simulink model "Test_Byte_Demultiplexer_1_to_4"  (Simulink 8.1)
settings: Solver=ode45  StartTime=0.0  StopTime=len  RelTol=1e-3
libraries: Byte_Demultiplexers_Lib x1, commutil2 x1
settings Model: Creator=N  LastModifiedBy=uzivatel
settings DataIOCC: LimitDataPoints=off  SignalLoggingSaveFormat=Dataset
settings OptimizationCC: ExpressionDepthLimit=128
settings DebuggingCC: UnderspecifiedInitializationDetection=Simplified  MergeDetectMultiDrivingBlocksExec=error  SolverPrmCheckMsg=none  FcnCallInpInsideContextMsg=EnableAllAsError  FrameProcessingCompatibilityMsg=error  StateNameClashWarn=none
settings HardwareCC: ProdBitPerPointer=64  ProdLargestAtomicFloat=Float  ProdIntDivRoundTo=Zero  ProdEndianess=LittleEndian  ProdHWDeviceType=Intel->x86-64 (Windows64)
settings ModelReferenceCC: PropagateSignalLabelsOutOfModel=on
settings GRTTargetCC: CodeReplacementLibrary=None  CombineOutputUpdateFcns=on  CPPClassGenCompliant=on  GRTInterface=off

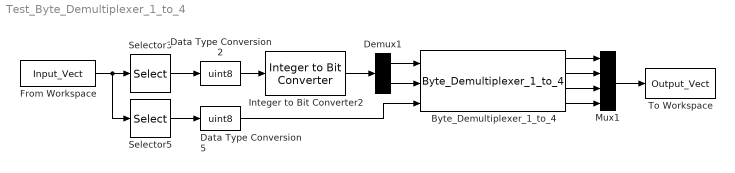
== system Test_Byte_Demultiplexer_1_to_4 ==
  Byte_Demultiplexer_1_to_4 : Byte_Demultiplexers_Lib/Byte_Demultiplexers_Lib/Byte_Demultiplexer_1_to_4
  Data Type Conversion2 : DataTypeConversion  OutDataTypeStr=uint8
  Data Type Conversion5 : DataTypeConversion  OutDataTypeStr=uint8
  Demux1 : Demux  Outputs=2
  From Workspace : FromWorkspace  VariableName=Input_Vect  SampleTime=1  Interpolate=off  OutputAfterFinalValue=Holding final value
  Integer to Bit Converter2 : commutil2/Integer to Bit Converter  nbits=2  signedInputValues=Unsigned  bitOrder=MSB first  outDtype=boolean
  Mux1 : Mux
  Selector3 : Selector  IndexMode=Zero-based  InputPortWidth=2  SampleTime=1  IndexOptions=Index vector (dialog)  Indices=0  OutputSizes=1
  Selector5 : Selector  IndexMode=Zero-based  InputPortWidth=2  IndexOptions=Index vector (dialog)  Indices=1  OutputSizes=1
  To Workspace : ToWorkspace  VariableName=Output_Vect  SampleTime=1
  wires:
  Integer to Bit Converter2/1 -> Demux1/1
  Selector3/1 -> Data Type Conversion2/1
  Data Type Conversion2/1 -> Integer to Bit Converter2/1
  From Workspace/1 -> Selector5/1, Selector3/1
  Demux1/1 -> Byte_Demultiplexer_1_to_4/1
  Demux1/2 -> Byte_Demultiplexer_1_to_4/2
  Selector5/1 -> Data Type Conversion5/1
  Data Type Conversion5/1 -> Byte_Demultiplexer_1_to_4/3
  Mux1/1 -> To Workspace/1
  Byte_Demultiplexer_1_to_4/1 -> Mux1/1
  Byte_Demultiplexer_1_to_4/2 -> Mux1/2
  Byte_Demultiplexer_1_to_4/3 -> Mux1/3
  Byte_Demultiplexer_1_to_4/4 -> Mux1/4
